simulink model "shuixiang_pid"  (R2013a)
settings: Solver=ode3  StartTime=0.0  StopTime=10.0  FixedStep=0.001  RelTol=1e-7
values from neighbouring files (symbols this model uses):
  kd = x(i,3)    [ABCPID.m]    (also in WPSO_PID.m; cpso_pid1.m)
  ki = x(i,2)    [ABCPID.m]    (also in WPSO_PID.m; cpso_pid1.m)
  kp = x(i,1)    [ABCPID.m]    (also in WPSO_PID.m; cpso_pid1.m)
settings Model: Creator=Administrator  LastModifiedBy=sjp
settings SolverCC: ZeroCrossControl=DisableAll
settings DebuggingCC: SolverPrmCheckMsg=none

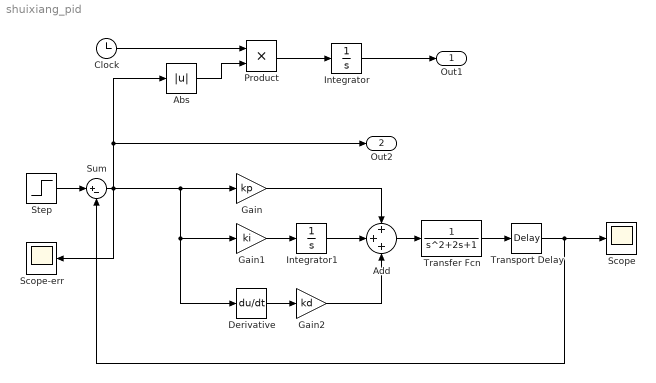
== system shuixiang_pid ==
  "              Add" : Sum  Inputs=+++
  Abs : Abs
  Clock : Clock
  Derivative : Derivative
  Gain : Gain  Gain=kp
  Gain1 : Gain  Gain=ki
  Gain2 : Gain  Gain=kd
  Integrator : Integrator
  Integrator1 : Integrator
  Product : Product
  Scope : Scope
      settings: TimeRange=5  YMin=0  YMax=1.5  SaveName=y
  Scope-err : Scope
      settings: TimeRange=5  YMin=0  YMax=1.5  SaveName=err_out
  Step : Step  Time=0  SampleTime=0
  Sum : Sum  Inputs=|+-
  Transfer Fcn : TransferFcn
  Transport Delay : TransportDelay  DelayTime=0.5
  Out1 : Outport
  Out2 : Outport  Port=2
  wires:
  Step/1 -> Sum/1
  Integrator/1 -> Out1/1
  Transfer Fcn/1 -> Transport Delay/1
  Product/1 -> Integrator/1
  Clock/1 -> Product/1
  Abs/1 -> Product/2
  "              Add"/1 -> Transfer Fcn/1
  Integrator1/1 -> "              Add"/2
  Gain2/1 -> "              Add"/3
  Derivative/1 -> Gain2/1
  Gain1/1 -> Integrator1/1
  Gain/1 -> "              Add"/1
  Transport Delay/1 -> Scope/1, Sum/2
  Sum/1 -> Scope-err/1, Gain/1, Gain1/1, Derivative/1, Out2/1, Abs/1
